simulink model "simulink_Example"  (R2020a)
settings: Solver=ode4  StartTime=0.0  StopTime=10.0  FixedStep=0.01  RelTol=1e-3
settings Model: Creator=Juan Augusto Paredes  LastModifiedBy=Juan Augusto Paredes

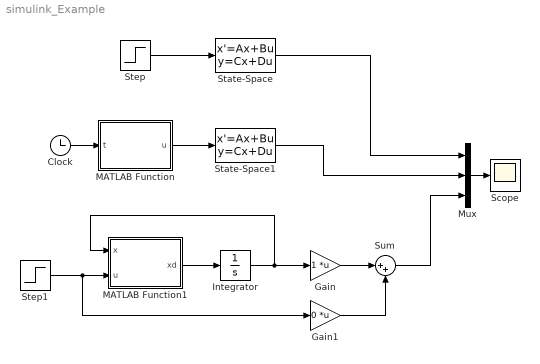
== system simulink_Example ==
  Clock : Clock
  Gain : Gain  Multiplication=Matrix(K*u)
  Gain1 : Gain  Gain=0  Multiplication=Matrix(K*u)
  Integrator : Integrator  InitialCondition=2
  MATLAB Function : MATLAB Function  TreatAsAtomicUnit=on
  MATLAB Function1 : MATLAB Function  TreatAsAtomicUnit=on
  Mux : Mux  Inputs=3
  Scope : Scope
  State-Space : StateSpace  A=-1  D=0  InitialCondition=2
  State-Space1 : StateSpace  A=-1  D=0  InitialCondition=2
  Step : Step  After=5  SampleTime=0
  Step1 : Step  After=5  SampleTime=0
  Sum : Sum  Inputs=|++
  wires:
  Clock/1 -> MATLAB Function/1(t)
  Step/1 -> State-Space/1
  MATLAB Function/1(u) -> State-Space1/1
  Step1/1 -> Gain1/1, MATLAB Function1/2(u)
  MATLAB Function1/1(xd) -> Integrator/1
  Integrator/1 -> Gain/1, MATLAB Function1/1(x)
  Gain/1 -> Sum/1
  Gain1/1 -> Sum/2
  State-Space/1 -> Mux/1
  State-Space1/1 -> Mux/2
  Sum/1 -> Mux/3
  Mux/1 -> Scope/1

== matlab function simulink_Example/MATLAB Function ==
  data: t input; u output
function u = stepFun(t)
    u = 5.*(t>=1);
end

== matlab function simulink_Example/MATLAB Function1 ==
  data: x input; u input; xd output
function xd = odefun(x, u)

    A = -1;
    B = 1;

    xd = A*x + B*u;

end
